simulink model "TestLpe"  (R2015b)
settings: Solver=VariableStepAuto  StartTime=0.0  StopTime=60  RelTol=1e-3
InitFcn:
  | load tfwt_00_run_01.mat
libraries: Px4Library x1
settings Model: Creator=jban039  LastModifiedBy=jban039

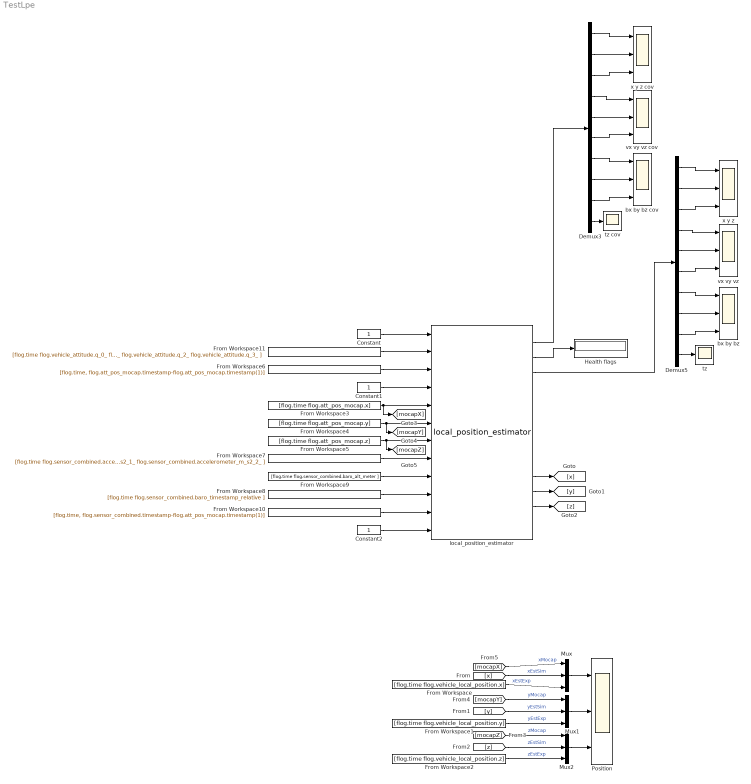
== system TestLpe ==
  Constant : Constant
  Constant1 : Constant
  Constant2 : Constant
  Demux3 : Demux  Outputs=10
  Demux5 : Demux  Outputs=10
  From Workspace : FromWorkspace  VariableName=[flog.time flog.vehicle_local_position.x]  SampleTime=0  Interpolate=off  OutputAfterFinalValue=Holding final value
  From Workspace1 : FromWorkspace  VariableName=[flog.time flog.vehicle_local_position.y]  SampleTime=0  Interpolate=off  OutputAfterFinalValue=Holding final value
  From Workspace10 : FromWorkspace  VariableName=[flog.time, flog.sensor_combined.timestamp-flog.att_pos_mocap.timestamp(1)]  SampleTime=0  Interpolate=off  OutputAfterFinalValue=Holding final value
  From Workspace11 : FromWorkspace  VariableName=[flog.time flog.vehicle_attitude.q_0_ flog.vehicle_attitude.q_1_ flog.vehicle_attitude.q_2_ flog.vehicle_attitude.q_3_ ]  SampleTime=0  Interpolate=off  OutputAfterFinalValue=Holding final value
  From Workspace2 : FromWorkspace  VariableName=[flog.time flog.vehicle_local_position.z]  SampleTime=0  Interpolate=off  OutputAfterFinalValue=Holding final value
  From Workspace3 : FromWorkspace  VariableName=[flog.time flog.att_pos_mocap.x]  SampleTime=0  Interpolate=off  OutputAfterFinalValue=Holding final value
  From Workspace4 : FromWorkspace  VariableName=[flog.time flog.att_pos_mocap.y]  SampleTime=0  Interpolate=off  OutputAfterFinalValue=Holding final value
  From Workspace5 : FromWorkspace  VariableName=[flog.time flog.att_pos_mocap.z]  SampleTime=0  Interpolate=off  OutputAfterFinalValue=Holding final value
  From Workspace6 : FromWorkspace  VariableName=[flog.time, flog.att_pos_mocap.timestamp-flog.att_pos_mocap.timestamp(1)]  SampleTime=0  Interpolate=off  OutputAfterFinalValue=Holding final value
  From Workspace7 : FromWorkspace  VariableName=[flog.time flog.sensor_combined.accelerometer_m_s2_0_ flog.sensor_combined.accelerometer_m_s2_1_ flog.sensor_combined.accelerometer_m_s2_2_ ]  SampleTime=0  Interpolate=off  OutputAfterFinalValue=Holding final value
  From Workspace8 : FromWorkspace  VariableName=[flog.time flog.sensor_combined.baro_timestamp_relative ]  SampleTime=0  Interpolate=off  OutputAfterFinalValue=Holding final value
  From Workspace9 : FromWorkspace  VariableName=[flog.time flog.sensor_combined.baro_alt_meter ]  SampleTime=0  Interpolate=off  OutputAfterFinalValue=Holding final value
  Health flags : Display
  Mux : Mux  Inputs=3
  Mux1 : Mux  Inputs=3
  Mux2 : Mux  Inputs=3
  Position : Scope  NumInputPorts=3
  bx by bz : Scope  NumInputPorts=3
  bx by bz cov : Scope  NumInputPorts=3
  local_position_estimator : Px4Library/local_position_estimator  LPE_SAMPLING_PERIOD=0.01  LPE_ACC_XY=0.012  LPE_ACC_Z=0.020  LPE_BAR_Z=3.0  LPE_EPH_MAX=3.0  LPE_EPV_MAX=5.0  LPE_FAKE_ORIGIN=0.0  LPE_FGYRO_HP=0.0010  LPE_FLW_OFF_Z=0.0  LPE_FLW_QMIN=150.0  LPE_FLW_R=7.0  LPE_FLW_RR=7.0  LPE_FLW_SCALE=1.300  LPE_GPS_DELAY=0.290  LPE_GPS_VXY=0.250  LPE_GPS_VZ=0.250  LPE_GPS_XY=1.000  LPE_GPS_Z=3.0  LPE_LAND_VXY=0.050  LPE_LAND_Z=0.030  LPE_LAT=47.398  LPE_LDR_OFF_Z=0.0  LPE_LDR_Z=0.030  LPE_LON=8.546  LPE_PN_B=0.0010  LPE_PN_P=0.100  LPE_PN_T=0.0010  LPE_PN_V=0.100  LPE_SNR_OFF_Z=0.0  LPE_SNR_Z=0.050  LPE_T_MAX_GRADE=1.000  LPE_VIC_P=0.0010  LPE_VIS_DELAY=0.100  LPE_VIS_XY=0.100  LPE_VIS_Z=0.500  LPE_VXY_PUB=0.300  LPE_X_LP=5.0  LPE_Z_PUB=1.000  LPE_FUSION=193  Barometer=on  GPS=off  LIDAR=off  Flow=off  Sonar=off  Vision=off  Mocap=on  Land=on
  tz : Scope
  tz cov : Scope
  vx vy vz : Scope  NumInputPorts=3
  vx vy vz cov : Scope  NumInputPorts=3
  x y z : Scope  NumInputPorts=3
  x y z cov : Scope  NumInputPorts=3
  wires:
  Mux1/1 -> Position/2
  Mux/1 -> Position/1
  Mux2/1 -> Position/3
  Demux5/2 -> x y z/2
  Demux5/1 -> x y z/1
  Demux5/3 -> x y z/3
  Demux5/4 -> vx vy vz/1
  Demux5/5 -> vx vy vz/2
  Demux5/6 -> vx vy vz/3
  Demux5/7 -> bx by bz/1
  Demux5/8 -> bx by bz/2
  Demux5/9 -> bx by bz/3
  Demux5/10 -> tz/1
  local_position_estimator/3 -> Demux5/1
  Demux3/2 -> x y z cov/2
  Demux3/1 -> x y z cov/1
  Demux3/3 -> x y z cov/3
  Demux3/4 -> vx vy vz cov/1
  Demux3/5 -> vx vy vz cov/2
  Demux3/6 -> vx vy vz cov/3
  Demux3/7 -> bx by bz cov/1
  Demux3/8 -> bx by bz cov/2
  Demux3/9 -> bx by bz cov/3
  Demux3/10 -> tz cov/1
  local_position_estimator/1 -> Demux3/1
  local_position_estimator/2 -> Health flags/1
  local_position_estimator/10 -> [x]
  local_position_estimator/11 -> [y]
  local_position_estimator/12 -> [z]
  From Workspace1/1 -> Mux1/3  "yEstExp"
  From Workspace2/1 -> Mux2/3  "zEstExp"
  From Workspace/1 -> Mux/3  "xEstExp"
  [x] -> Mux/2  "xEstSim"
  [y] -> Mux1/2  "yEstSim"
  [z] -> Mux2/2  "zEstSim"
  From Workspace3/1 -> local_position_estimator/5, [mocapX]
  From Workspace5/1 -> local_position_estimator/7, [mocapZ]
  From Workspace4/1 -> local_position_estimator/6, [mocapY]
  From Workspace6/1 -> local_position_estimator/3
  Constant/1 -> local_position_estimator/1
  [mocapX] -> Mux/1  "xMocap"
  [mocapY] -> Mux1/1  "yMocap"
  [mocapZ] -> Mux2/1  "zMocap"
  Constant1/1 -> local_position_estimator/4
  From Workspace7/1 -> local_position_estimator/8
  From Workspace8/1 -> local_position_estimator/10
  From Workspace9/1 -> local_position_estimator/9
  From Workspace10/1 -> local_position_estimator/11
  Constant2/1 -> local_position_estimator/12
  From Workspace11/1 -> local_position_estimator/2
